simulink subsystem "Subsystem_Obstaculos_Leds"  (R2023b)
settings: Solver=VariableStepAuto  StartTime=0.0  StopTime=10.0  RelTol=1e-3
settings Model: Creator=Alberto  LastModifiedBy=Gonzalo

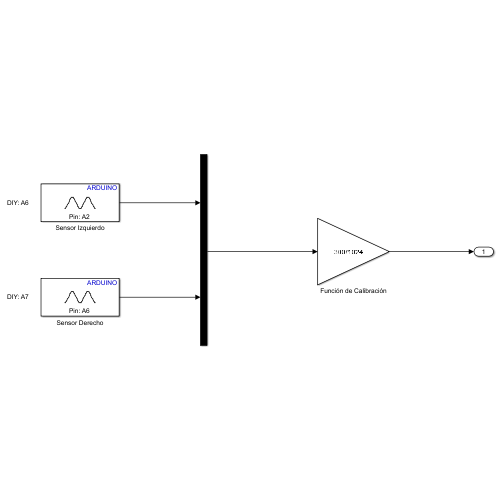
[thumbnail: Simulink's stored preview of the top-level diagram]
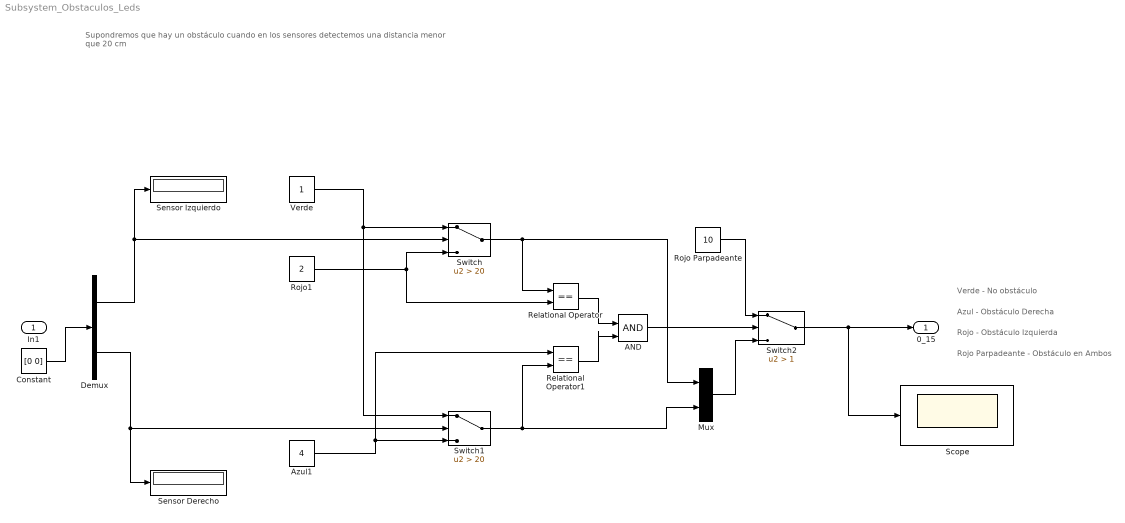
== system Subsystem_Obstaculos_Leds ==
  note: Verde - No obstáculo
  note: Azul - Obstáculo Derecha
  note: Rojo - Obstáculo Izquierda
  note: Rojo Parpadeante - Obstáculo en Ambos
  note: Supondremos que hay un obstáculo cuando en los sensores detectemos una distancia menor que 20 cm
  In1 : Inport
  AND : Logic  IconShape=distinctive  AllPortsSameDT=off  OutDataTypeStr=boolean
  Azul1 : Constant  Value=4
  Constant : Constant  Value=[0 0]
  Demux : Demux  Outputs=2
  Mux : Mux  Inputs=2
  Relational Operator : RelationalOperator  Operator===  OutDataTypeStr=boolean  RndMeth=Simplest  InputSameDT=off
  Relational Operator1 : RelationalOperator  Operator===  OutDataTypeStr=boolean  RndMeth=Simplest  InputSameDT=off
  Rojo Parpadeante : Constant  Value=10
  Rojo1 : Constant  Value=2
  Scope : Scope
  Sensor Derecho : Display
  Sensor Izquierdo : Display
  Switch : Switch  Criteria=u2 > Threshold  Threshold=20  SaturateOnIntegerOverflow=off  InputSameDT=off
  Switch1 : Switch  Criteria=u2 > Threshold  Threshold=20  SaturateOnIntegerOverflow=off  InputSameDT=off
  Switch2 : Switch  Criteria=u2 > Threshold  Threshold=1  SaturateOnIntegerOverflow=off  InputSameDT=off
  Verde : Constant
  0_15 : Outport
  wires:
  Demux/2 -> Sensor Derecho/1, Switch1/2
  Demux/1 -> Switch/2, Sensor Izquierdo/1
  Verde/1 -> Switch/1, Switch1/1
  Rojo1/1 -> Switch/3, Relational Operator/2
  Azul1/1 -> Switch1/3, Relational Operator1/1
  Switch/1 -> Relational Operator/1, Mux/1
  Switch1/1 -> Relational Operator1/2, Mux/2
  Relational Operator/1 -> AND/1
  Relational Operator1/1 -> AND/2
  AND/1 -> Switch2/2
  Switch2/1 -> 0_15/1, Scope/1
  Rojo Parpadeante/1 -> Switch2/1
  Mux/1 -> Switch2/3
  Constant/1 -> Demux/1
